simulink library "Isolated_Cover"  (Simulink 8.2)
settings: Solver=ode45  StartTime=0.0  StopTime=10.0  RelTol=1e-3
settings Model: Creator=lena.frank  LastModifiedBy=drhf

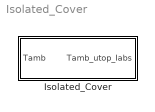
== system Isolated_Cover ==
  Isolated_Cover : Subsystem  mask(isolated cover){u=0.6}
      mask prompts: u "loss coefficient of isolation [W/(m²*K)]"
      mask help: This is a surface-model for ground storages. It describes the absorption of solar radiation and the heat losses by wind.
      mask Help: web(fullfile(path_carnot('help'),'Isolated_Cover.html'),'-helpbrowser')

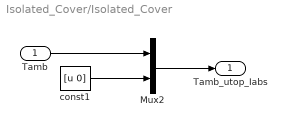
== system Isolated_Cover/Isolated_Cover ==
  Tamb : Inport
  Mux2 : Mux  Inputs=2
  const1 : Constant  Value=[u 0]
  Tamb_utop_Iabs : Outport
  wires:
  Tamb/1 -> Mux2/1
  const1/1 -> Mux2/2
  Mux2/1 -> Tamb_utop_Iabs/1
